simulink model "sampleModel1631_1"  (R2023a)
settings: Solver=VariableStepAuto  StartTime=0.0  StopTime=10.0  RelTol=1e-3
libraries: simulink x2, hdlsllib x2
settings Model: Creator=user1  LastModifiedBy=user1

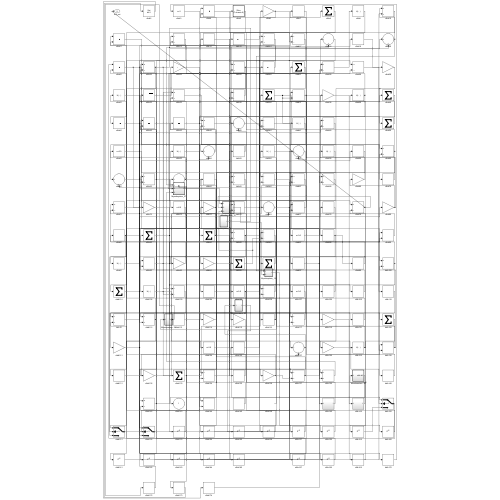
[thumbnail: Simulink's stored preview of the top-level diagram]
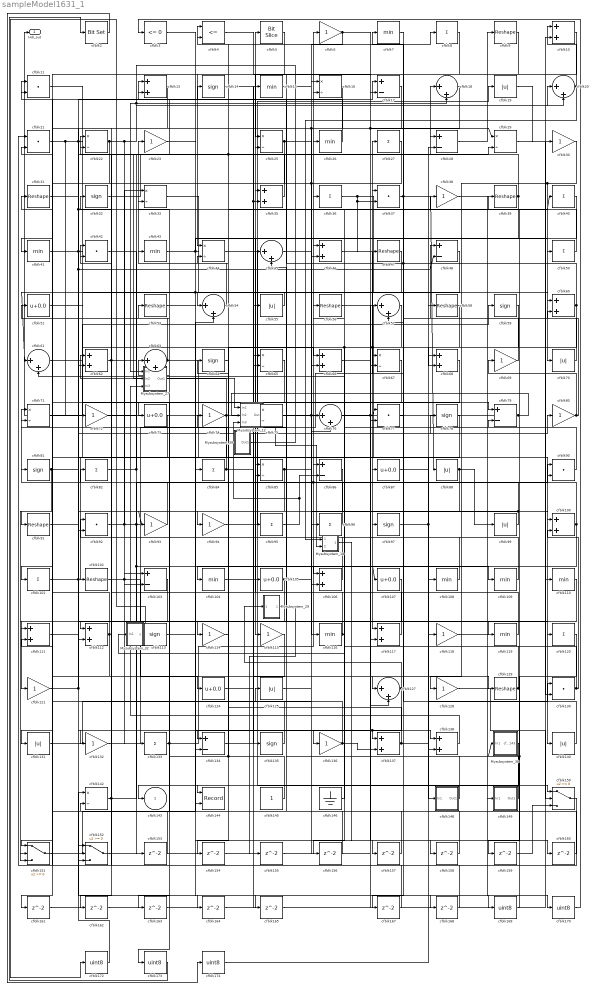
== system sampleModel1631_1 ==
  Mysubsystem_12 : Subsystem  TreatAsAtomicUnit=on  RTWFcnName=Mysubsystem_12
      settings: RTWFcnNameOpts=User specified  RTWFileNameOpts=Use function name
  Mysubsystem_18 : Subsystem  TreatAsAtomicUnit=on  RTWFcnName=Mysubsystem_18
      settings: RTWFcnNameOpts=User specified  RTWFileNameOpts=Use function name
  Mysubsystem_27 : Subsystem  TreatAsAtomicUnit=on  RTWFcnName=Mysubsystem_27
      settings: RTWFcnNameOpts=User specified  RTWFileNameOpts=Use function name
  Mysubsystem_29 : Subsystem  TreatAsAtomicUnit=on  RTWFcnName=Mysubsystem_29
      settings: RTWFcnNameOpts=User specified  RTWFileNameOpts=Use function name
  Mysubsystem_32 : Subsystem  TreatAsAtomicUnit=on  RTWFcnName=Mysubsystem_32
      settings: RTWFcnNameOpts=User specified  RTWFileNameOpts=Use function name
  Mysubsystem_38 : Subsystem  TreatAsAtomicUnit=on  RTWFcnName=Mysubsystem_38
      settings: RTWFcnNameOpts=User specified  RTWFileNameOpts=Use function name
  Mysubsystem_39 : Subsystem  TreatAsAtomicUnit=on  RTWFcnName=Mysubsystem_39
      settings: RTWFcnNameOpts=User specified  RTWFileNameOpts=Use function name
  cfblk{10,13,35,46,60,62,66,68,100,106,111..112,117,137..138} (15 alike) : Sum  OutDataTypeStr=uint8
  cfblk{8,27,36,40,50,82,84,95..96,101,120,133} (12 alike) : Sum  Inputs=+  OutDataTypeStr=uint8
  cfblk{9,31,39,47,53,56,58,91,102,129} (10 alike) : Reshape
  cfblk{17,28,48,79,86,103,134} (7 alike) : Sum  Inputs=+-  OutDataTypeStr=uint8
  cfblk{7,15,26,41,43,104,108..110,116,119} (11 alike) : MinMax  OutDataTypeStr=uint8
  cfblk{51,73,87,105,107,124} (6 alike) : Bias  Bias=0.0  SaturateOnIntegerOverflow=off
  cfblk{11,21,37,42,77,90,92,130} (8 alike) : DotProduct  OutDataTypeStr=uint8
  cfblk{14,32,59,64,78,81,97,113,135} (9 alike) : Signum
  cfblk{6,23,30,38,69,72,74,80,93..94,114..115,118,121,128,132,136} (17 alike) : Gain  OutDataTypeStr=uint8
  cfblk{19,55,70,88,99,125,131,140} (8 alike) : Abs  OutDataTypeStr=uint8  SaturateOnIntegerOverflow=off
  cfblk{18,20,45,54,57,61,63,76,127} (9 alike) : Sum  Inputs=|++  OutDataTypeStr=uint8
  cfblk{16,22,25,29,33,44,65,67,71,75,85,142} (12 alike) : Product  Inputs=*/  OutDataTypeStr=uint8  RndMeth=Zero  SaturateOnIntegerOverflow=on
  cfblk144 : Record  FileSettingsInternal="{\"entries\":[{\"content\":{\"excelSettings\":{\"content\":{},\"type\":\"Streamout.ExcelSettings\"}},\"type\":\"Streamout.FileSettingStorage\",\"uuid\":\"\"}],\"packageUris\":[\"http:\\/\\/schema.mathworks.com\\/mf0\\/streamout_blocks\\/R2020a\"],\"version\":\"1.0\"}"  Layout=[1 1]  SignalsInternal="{\"entries\":[{\"content\":{\"signals\":[{\"content\":{\"blockPath\":[],\"dimensions\":[1],\"domain\":\"\",\"lineColor\":\"#a2142f\",\"plots\":[1],\"port\":1,\"signalID\":30493,\"signalName\":\"cfblk64\"},\"type\":\"RecordBlkView.Signal\",\"uuid\":\"\"},{\"content\":{\"blockPath\":[],\"dimensions\":[1],\"domain\":\"\",\"lineColor\":\"#139fff\",\"plots\":[1],\"port\":2,\"signalID\":30496,\"signalName\":\"cfblk40\"},\"type\":\"RecordBlkView.Signal\",\"uuid\":\"\"}]},\"type\":\"RecordBlkView.InputSignals\",\"uuid\":\"\"}],\"packageUris\":[\"http:\\/\\/schema.mathworks.com\\/mf0\\/streamout_blocks\\/R2020a\"],\"version\":\"1.0\"}"  VisualizationBindings="{\"xyplotplugin\":{\"info\":[{\"series\":[{\"bindingParametersList\":[{\"parameter\":\"X-Axis\",\"signalID\":30493,\"signalName\":\"cfblk64\"},{\"parameter\":\"Y-Axis\",\"signalID\":30496,\"signalName\":\"cfblk40\"}],\"seriesID\":15237}],\"subplotID\":1}]}}"  CompatibilityTag=XY  st=-1
  cfblk145 : Constant  OutDataTypeStr=uint8  SampleTime=-1
  cfblk146 : Ground
  cfblk148 : Subsystem
      settings: LibrarySourceBlock=|
      | hdlsllib/Ports &
      | Subsystems/Subsystem
  cfblk149 : Subsystem
      settings: LibrarySourceBlock=|
      | hdlsllib/Ports &
      | Subsystems/Subsystem
  cfblk150 : Switch  OutDataTypeStr=uint8  SaturateOnIntegerOverflow=off  InputSameDT=off
  cfblk151 : Switch  OutDataTypeStr=uint8  SaturateOnIntegerOverflow=off  InputSameDT=off
  cfblk152 : Switch  OutDataTypeStr=uint8  SaturateOnIntegerOverflow=off  InputSameDT=off
  cfblk{153..165,167..168} (15 alike) : Delay  SampleTime=1
  cfblk{169..170,172..174} (5 alike) : DataTypeConversion  OutDataTypeStr=uint8  SaturateOnIntegerOverflow=off  RndMeth=Floor
  cfblk2 : simulink/Logic and Bit Operations/Bit Set  iBit=0
      settings: LibrarySourceBlock=|
      | hdlsllib/Logic and Bit
      | Operations/Bit Set
  cfblk3 : hdlsllib/Logic and Bit Operations/Compare To Zero  relop=<=  OutDataTypeStr=uint8
  cfblk4 : RelationalOperator  Operator=<=  OutDataTypeStr=boolean  InputSameDT=off
  cfblk5 : hdlsllib/Logic and Bit Operations/Bit Slice  lidx=7  ridx=0
  cfblk143 : Outport  OutDataTypeStr=uint8  VectorParamsAs1DForOutWhenUnconnected=off
  Hdl_out : Outport  Port=2  OutDataTypeStr=uint8
  wires:
  cfblk55/1 -> cfblk54/1
  cfblk17/1 -> cfblk114/1
  cfblk60/1 -> Mysubsystem_32/1(In1), cfblk94/1, cfblk117/1, cfblk11/1, cfblk37/1
  cfblk127/1 -> Mysubsystem_29/1(In1), cfblk137/1, cfblk152/3
  cfblk46/1 -> cfblk87/1
  cfblk48/1 -> cfblk61/1, cfblk134/2
  cfblk133/1 -> cfblk6/1, cfblk163/1
  cfblk37/1 -> cfblk88/1, cfblk167/1
  cfblk21/1 -> cfblk73/1, cfblk120/1, cfblk72/1
  cfblk51/1 -> cfblk66/1
  cfblk93/1 -> cfblk71/1
  cfblk53/1 -> cfblk109/1
  cfblk107/1 -> cfblk121/1
  cfblk44/1 -> cfblk150/1
  cfblk132/1 -> cfblk27/1
  cfblk57/1 -> cfblk106/1
  cfblk117/1 -> cfblk5/1
  cfblk113/1 -> cfblk138/1
  cfblk54/1 -> cfblk23/1
  cfblk56/1 -> cfblk140/1
  cfblk102/1 -> cfblk124/1, cfblk103/2
  cfblk94/1 -> cfblk19/1
  cfblk32/1 -> cfblk18/1
  cfblk90/1 -> cfblk61/2
  cfblk39/1 -> cfblk115/1, cfblk22/1
  cfblk136/1 -> cfblk81/1, cfblk137/2
  cfblk10/1 -> cfblk25/1
  cfblk140/1 -> cfblk35/1
  cfblk87/1 -> cfblk68/1
  cfblk80/1 -> cfblk69/1, cfblk60/2
  cfblk151/1 -> cfblk54/2
  cfblk92/1 -> cfblk15/1, cfblk85/2, cfblk33/1, cfblk133/1
  cfblk72/1 -> cfblk113/1
  cfblk65/1 -> cfblk151/1
  cfblk84/1 -> cfblk135/1, cfblk71/2
  cfblk131/1 -> cfblk76/1
  cfblk11/1 -> cfblk84/1
  cfblk35/1 -> cfblk13/1
  cfblk148/1(Out1) -> cfblk95/1
  cfblk63/1 -> cfblk108/1, cfblk11/2
  cfblk59/1 -> cfblk68/2
  cfblk105/1 -> cfblk20/2, cfblk154/1
  cfblk15/1 -> cfblk8/1
  cfblk150/1 -> cfblk21/1
  cfblk76/1 -> cfblk77/1, cfblk100/1
  cfblk26/1 -> cfblk13/2
  cfblk19/1 -> cfblk30/1
  cfblk41/1 -> cfblk105/1, cfblk164/1
  cfblk14/1 -> cfblk35/2, cfblk136/1
  cfblk77/1 -> cfblk7/1
  cfblk30/1 -> cfblk70/1, cfblk128/1
  cfblk28/1 -> cfblk9/1
  cfblk129/1 -> cfblk46/1, cfblk79/2
  cfblk135/1 -> cfblk125/1
  cfblk38/1 -> cfblk149/1(In1)
  cfblk43/1 -> cfblk116/1, cfblk50/1
  cfblk71/1 -> cfblk59/1
  cfblk149/1(Out1) -> cfblk75/2
  cfblk137/1 -> cfblk130/1, cfblk64/1
  cfblk3/1 -> cfblk169/1
  cfblk64/1 -> cfblk144/1
  cfblk128/1 -> cfblk150/2
  cfblk70/1 -> cfblk48/1
  cfblk109/1 -> cfblk42/1
  cfblk31/1 -> cfblk152/1
  cfblk20/1 -> Mysubsystem_18/1(In1), cfblk10/1
  cfblk5/1 -> cfblk41/1
  cfblk16/1 -> cfblk46/2, cfblk62/2
  cfblk121/1 -> cfblk26/1, cfblk48/2, cfblk165/1
  cfblk22/1 -> cfblk103/1, cfblk20/1, cfblk101/1
  cfblk134/1 -> cfblk55/1
  cfblk88/1 -> cfblk138/2, cfblk99/1
  cfblk95/1 -> Mysubsystem_12/3(In3), cfblk86/2
  cfblk78/1 -> cfblk102/1
  cfblk40/1 -> cfblk144/2
  cfblk58/1 -> cfblk104/1
  cfblk74/1 -> cfblk152/2, cfblk62/1
  cfblk115/1 -> cfblk131/1
  cfblk7/1 -> cfblk57/2
  cfblk75/1 -> cfblk97/1, cfblk29/2
  cfblk145/1 -> cfblk43/1, cfblk74/1
  cfblk106/1 -> cfblk63/1
  cfblk33/1 -> cfblk130/2
  cfblk85/1 -> cfblk132/1, cfblk78/1
  cfblk116/1 -> cfblk92/1, cfblk36/1
  cfblk8/1 -> cfblk44/1
  cfblk99/1 -> cfblk93/1, cfblk33/2
  cfblk104/1 -> cfblk127/1
  cfblk146/1 -> cfblk56/1
  cfblk108/1 -> cfblk82/1
  cfblk100/1 -> cfblk31/1, cfblk134/1
  cfblk124/1 -> cfblk65/1
  cfblk114/1 -> Mysubsystem_27/2(In2), cfblk14/1
  cfblk47/1 -> cfblk106/2
  cfblk13/1 -> cfblk112/1
  cfblk29/1 -> cfblk110/1
  cfblk25/1 -> cfblk96/1, cfblk65/2
  cfblk36/1 -> cfblk47/1, cfblk37/2, cfblk60/1
  cfblk73/1 -> cfblk91/1
  cfblk130/1 -> cfblk67/1, cfblk100/2
  cfblk142/1 -> cfblk32/1, cfblk90/1
  cfblk62/1 -> cfblk79/1, cfblk42/2
  cfblk69/1 -> cfblk25/2
  cfblk152/1 -> cfblk67/2
  cfblk119/1 -> cfblk53/1
  cfblk97/1 -> cfblk118/1, cfblk90/2
  cfblk82/1 -> cfblk119/1, cfblk107/1, cfblk28/1
  cfblk61/1 -> cfblk148/1(In1)
  cfblk45/1 -> cfblk117/2
  cfblk111/1 -> cfblk38/1
  cfblk27/1 -> cfblk66/2, cfblk112/2
  cfblk6/1 -> cfblk29/1, cfblk160/1, cfblk4/2
  cfblk125/1 -> cfblk17/1
  cfblk101/1 -> cfblk80/1, cfblk168/1
  cfblk9/1 -> cfblk45/1
  cfblk50/1 -> cfblk4/1
  cfblk91/1 -> cfblk40/1, cfblk16/2
  cfblk66/1 -> cfblk129/1
  cfblk112/1 -> cfblk51/1, cfblk161/1
  cfblk86/1 -> cfblk92/2
  cfblk96/1 -> cfblk44/2, cfblk86/1
  cfblk110/1 -> cfblk151/2
  cfblk18/1 -> cfblk111/1
  cfblk81/1 -> cfblk151/3, cfblk85/1
  cfblk4/1 -> cfblk17/2
  cfblk42/1 -> cfblk153/1
  cfblk153/1 -> cfblk142/2
  cfblk154/1 -> cfblk76/2
  cfblk155/1 -> cfblk127/2
  cfblk67/1 -> cfblk156/1
  cfblk156/1 -> cfblk21/2
  cfblk23/1 -> cfblk157/1
  cfblk157/1 -> cfblk16/1
  cfblk158/1 -> cfblk45/2
  cfblk120/1 -> cfblk159/1
  cfblk159/1 -> cfblk150/3
  cfblk160/1 -> cfblk63/2
  cfblk161/1 -> cfblk77/2
  cfblk103/1 -> cfblk162/1
  cfblk162/1 -> cfblk75/1
  cfblk163/1 -> cfblk10/2
  cfblk164/1 -> cfblk28/2
  cfblk165/1 -> cfblk57/1
  cfblk167/1 -> cfblk111/2
  cfblk168/1 -> cfblk22/2
  cfblk169/1 -> Mysubsystem_38/1(In1), cfblk39/1
  cfblk118/1 -> cfblk170/1
  cfblk170/1 -> cfblk3/1
  cfblk172/1 -> cfblk142/1
  cfblk68/1 -> cfblk173/1
  cfblk173/1 -> cfblk2/1
  cfblk2/1 -> cfblk174/1
  cfblk174/1 -> cfblk58/1
  cfblk79/1 -> Mysubsystem_12/2(In2), Hdl_out/1
  Mysubsystem_12/1(Out1) -> Mysubsystem_18/2(In2)
  Mysubsystem_18/1(Out1) -> cfblk158/1
  cfblk138/1 -> Mysubsystem_27/3(In3)
  Mysubsystem_27/1(Out1) -> Mysubsystem_12/1(In1)
  Mysubsystem_29/1(Out1) -> cfblk155/1
  Mysubsystem_32/1(y) -> cfblk172/1
  Mysubsystem_38/1(cfblk143) -> cfblk143/1
  Mysubsystem_39/1(Out1) -> Mysubsystem_27/1(In1), cfblk18/2

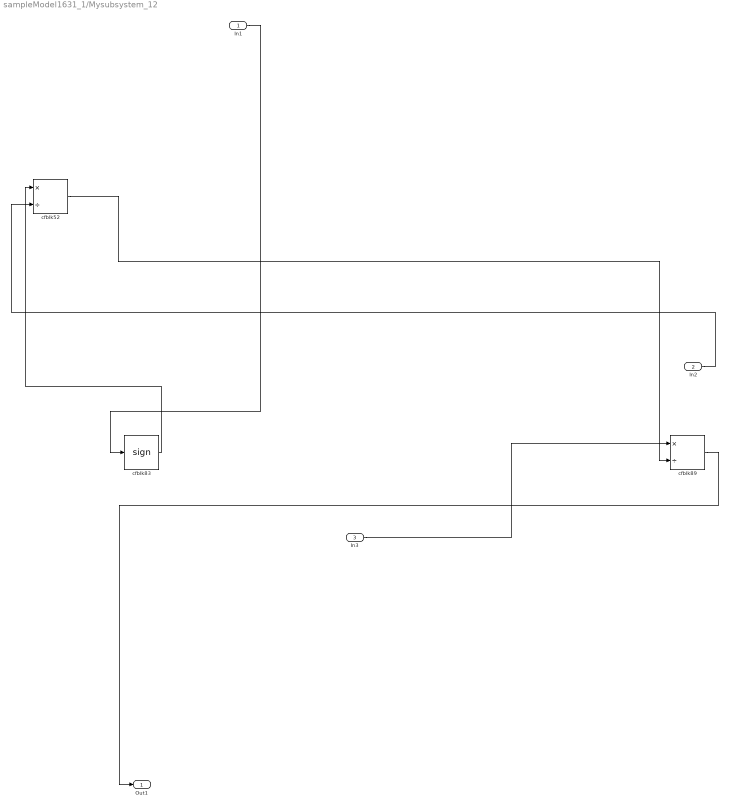
== system sampleModel1631_1/Mysubsystem_12 ==
  In1 : Inport
  In2 : Inport  Port=2
  In3 : Inport  Port=3
  cfblk52 : Product  Inputs=*/  RndMeth=Zero  SaturateOnIntegerOverflow=on
  cfblk83 : Signum
  cfblk89 : Product  Inputs=*/  RndMeth=Zero  SaturateOnIntegerOverflow=on
  Out1 : Outport
  wires:
  cfblk83/1 -> cfblk52/1
  In2/1 -> cfblk52/2
  In3/1 -> cfblk89/1
  cfblk52/1 -> cfblk89/2
  cfblk89/1 -> Out1/1
  In1/1 -> cfblk83/1

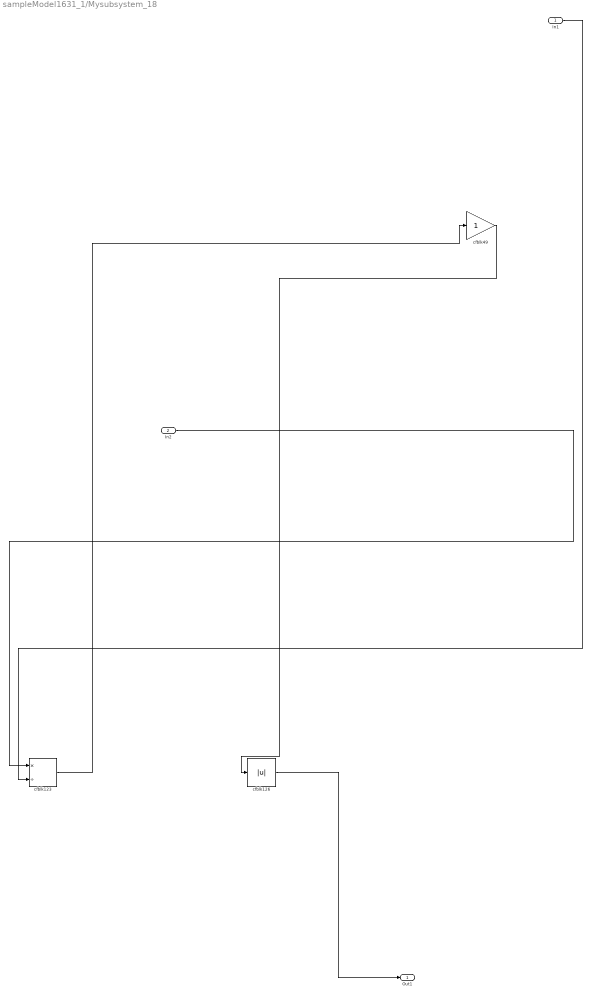
== system sampleModel1631_1/Mysubsystem_18 ==
  In1 : Inport
  In2 : Inport  Port=2
  cfblk123 : Product  Inputs=*/  RndMeth=Zero  SaturateOnIntegerOverflow=on
  cfblk126 : Abs  SaturateOnIntegerOverflow=off
  cfblk49 : Gain
  Out1 : Outport
  wires:
  In1/1 -> cfblk123/2
  cfblk123/1 -> cfblk49/1
  cfblk49/1 -> cfblk126/1
  In2/1 -> cfblk123/1
  cfblk126/1 -> Out1/1

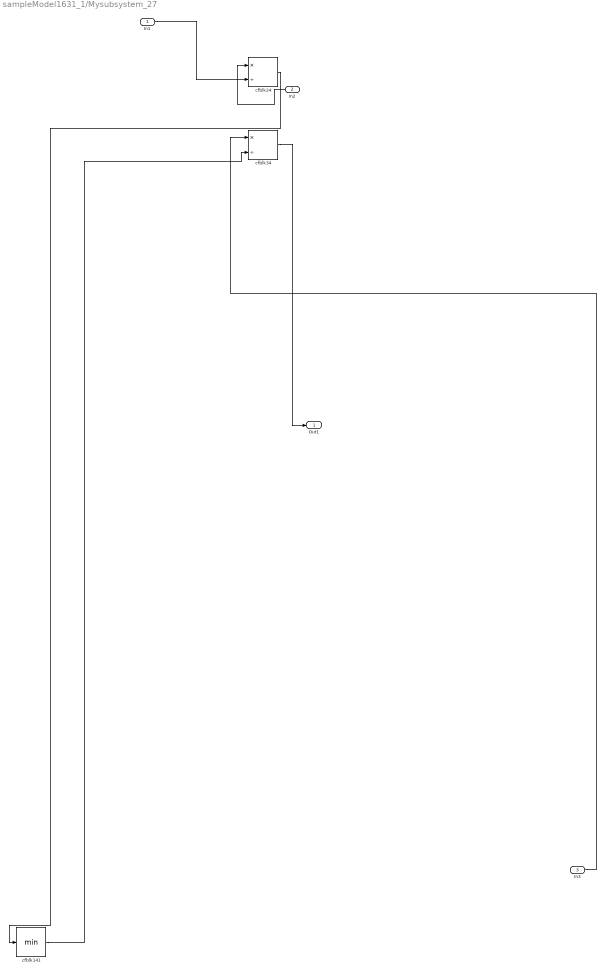
== system sampleModel1631_1/Mysubsystem_27 ==
  In1 : Inport
  In2 : Inport  Port=2
  In3 : Inport  Port=3
  cfblk141 : MinMax
  cfblk24 : Product  Inputs=*/  RndMeth=Zero  SaturateOnIntegerOverflow=on
  cfblk34 : Product  Inputs=*/  RndMeth=Zero  SaturateOnIntegerOverflow=on
  Out1 : Outport
  wires:
  cfblk34/1 -> Out1/1
  cfblk24/1 -> cfblk141/1
  cfblk141/1 -> cfblk34/2
  In1/1 -> cfblk24/2
  In2/1 -> cfblk24/1
  In3/1 -> cfblk34/1

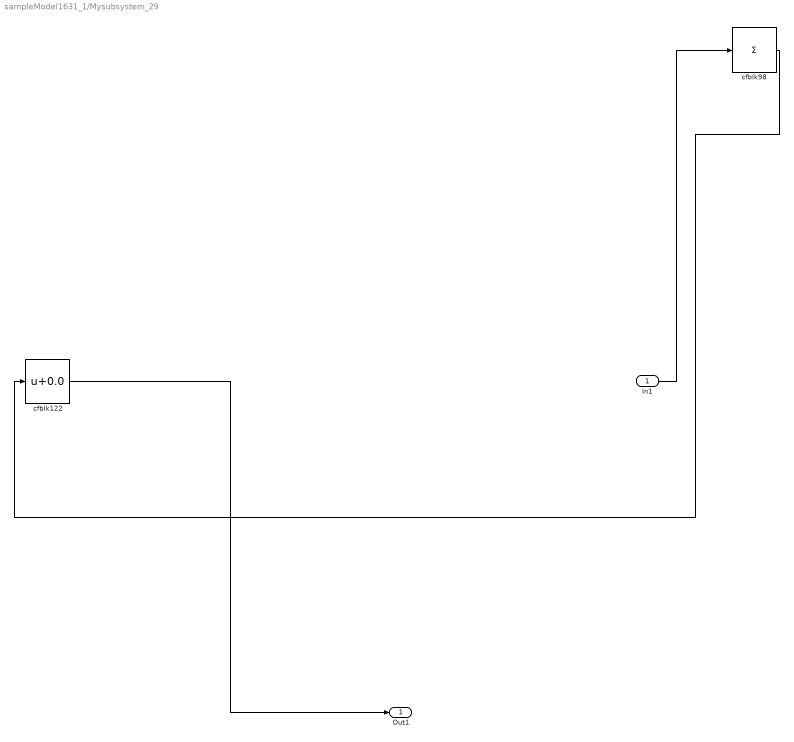
== system sampleModel1631_1/Mysubsystem_29 ==
  In1 : Inport
  cfblk122 : Bias  Bias=0.0  SaturateOnIntegerOverflow=off
  cfblk98 : Sum  Inputs=+
  Out1 : Outport
  wires:
  cfblk98/1 -> cfblk122/1
  In1/1 -> cfblk98/1
  cfblk122/1 -> Out1/1

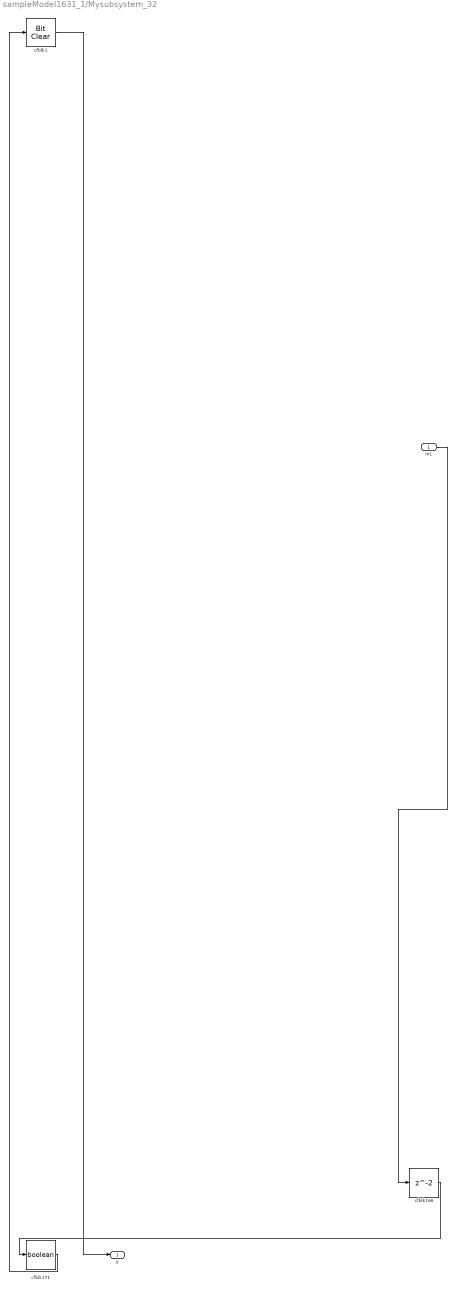
== system sampleModel1631_1/Mysubsystem_32 ==
  In1 : Inport
  cfblk1 : simulink/Logic and Bit Operations/Bit Clear  iBit=0
      settings: LibrarySourceBlock=|
      | hdlsllib/Logic and Bit
      | Operations/Bit Clear
  cfblk166 : Delay  SampleTime=1
  cfblk171 : DataTypeConversion  OutDataTypeStr=boolean  SaturateOnIntegerOverflow=off  RndMeth=Floor
  y : Outport
  wires:
  cfblk1/1 -> y/1
  In1/1 -> cfblk166/1
  cfblk166/1 -> cfblk171/1
  cfblk171/1 -> cfblk1/1

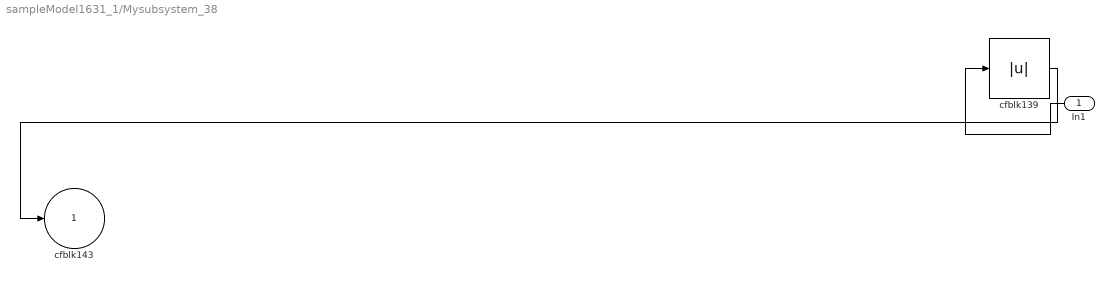
== system sampleModel1631_1/Mysubsystem_38 ==
  In1 : Inport
  cfblk139 : Abs  SaturateOnIntegerOverflow=off
  cfblk143 : Outport  VectorParamsAs1DForOutWhenUnconnected=off
  wires:
  cfblk139/1 -> cfblk143/1
  In1/1 -> cfblk139/1

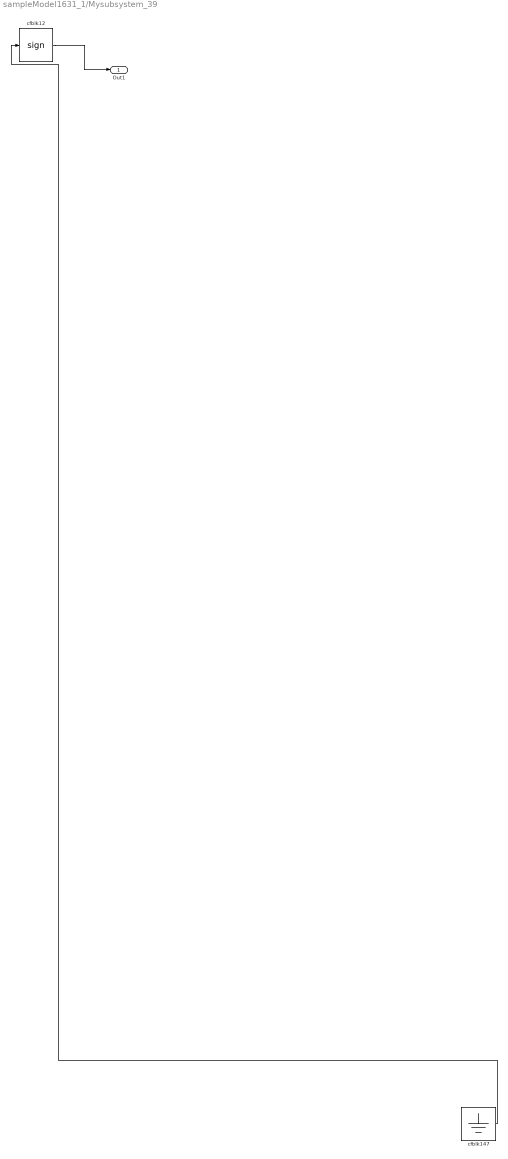
== system sampleModel1631_1/Mysubsystem_39 ==
  cfblk12 : Signum
  cfblk147 : Ground
  Out1 : Outport
  wires:
  cfblk147/1 -> cfblk12/1
  cfblk12/1 -> Out1/1

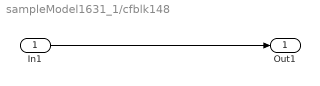
== system sampleModel1631_1/cfblk148 ==
  In1 : Inport
  Out1 : Outport
  wires:
  In1/1 -> Out1/1

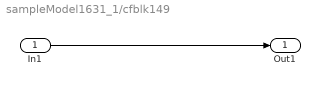
== system sampleModel1631_1/cfblk149 ==
  In1 : Inport
  Out1 : Outport
  wires:
  In1/1 -> Out1/1
